simulink model "motorcycle_LQR_with_integral_action"  (R2021a)
settings: Solver=VariableStepAuto  StartTime=0.0  StopTime=10  RelTol=1e-3
values from neighbouring files (symbols this model uses):
  A = [0 0;1 0]    [pole_placement.m]
  B = [1; 0]    [pole_placement.m]
  C = [0 1]    [pole_placement.m]
  k = place(A,B,P)    [pole_placement.m]
undefined symbols (not defined in the file or in its folder): L, L_tK
libraries: simulink x2
settings Model: Creator=martina.elle  LastModifiedBy=francesco

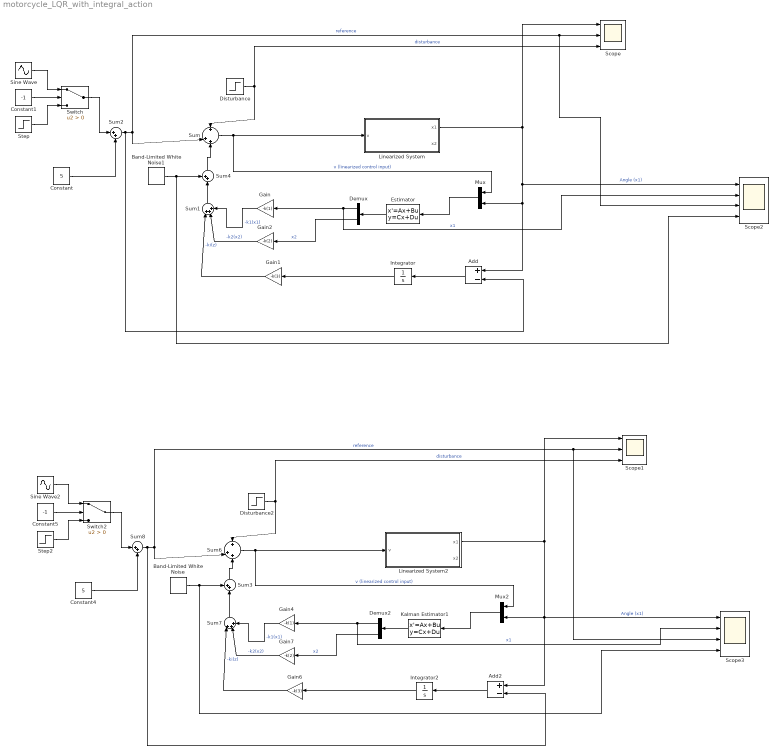
== system motorcycle_LQR_with_integral_action ==
  Add : Sum  Inputs=+-
  Add2 : Sum  Inputs=+-
  Band-Limited White Noise : simulink/Sources/Band-Limited White Noise  Cov=[1]  Ts=0.1  seed=[23341]
  Band-Limited White Noise1 : simulink/Sources/Band-Limited White Noise  Cov=[1]  Ts=0.1  seed=[23341]
  Constant : Constant  Value=5
  Constant1 : Constant  Value=-1
  Constant4 : Constant  Value=5
  Constant5 : Constant  Value=-1
  Demux : Demux  Outputs=2
  Demux2 : Demux  Outputs=2
  Disturbance : Step  After=3  SampleTime=0
  Disturbance2 : Step  After=3  SampleTime=0
  Estimator : StateSpace  A=A-L*C  B=[B L]  C=eye(2)  D=[0 0; 0 0]  InitialCondition=[0 0]  ParameterTunability=Unconstrained
  Gain : Gain  Gain=-k(1)
  Gain1 : Gain  Gain=-k(3)
  Gain2 : Gain  Gain=-k(2)
  Gain4 : Gain  Gain=-k(1)
  Gain6 : Gain  Gain=-k(3)
  Gain7 : Gain  Gain=-k(2)
  Integrator : Integrator  InitialCondition=-3
  Integrator2 : Integrator  InitialCondition=-3
  Kalman Estimator1 : StateSpace  A=A-L_tK*C  B=[B L_tK]  C=eye(2)  D=[0 0; 0 0]  InitialCondition=[0 0]  ParameterTunability=Unconstrained
  Linearized System : Subsystem
  Linearized System2 : Subsystem
  Mux : Mux  Inputs=2
  Mux2 : Mux  Inputs=2
  Scope : Scope  NumInputPorts=3
  Scope1 : Scope  NumInputPorts=3
  Scope2 : Scope  NumInputPorts=4
  Scope3 : Scope  NumInputPorts=4
  Sine Wave : Sin  Frequency=0.1  SampleTime=0
  Sine Wave2 : Sin  Frequency=0.1  SampleTime=0
  Step : Step  After=40  SampleTime=0
  Step2 : Step  After=40  SampleTime=0
  Sum : Sum  Inputs=+|++
  Sum1 : Sum  Inputs=|+++
  Sum2 : Sum  Inputs=|++
  Sum3 : Sum  Inputs=++|
  Sum4 : Sum  Inputs=++|
  Sum6 : Sum  Inputs=+|++
  Sum7 : Sum  Inputs=|+++
  Sum8 : Sum  Inputs=|++
  Switch : Switch  Criteria=u2 > Threshold
  Switch2 : Switch  Criteria=u2 > Threshold
  wires:
  Linearized System/1(x1) -> Mux/2, Add/1, Scope2/1, Scope/1  "Angle (x1)"
  Sum2/1 -> Sum/2, Scope2/3, Scope/2, Add/2  "reference"
  Sum/1 -> Linearized System/1("v "), Mux/1  "v (linearized control input)"
  Mux/1 -> Estimator/1
  Estimator/1 -> Demux/1
  Gain/1 -> Sum1/3  "-k1(x1)"
  Demux/2 -> Gain2/1  "x2"
  Gain2/1 -> Sum1/2  "-k2(x2)"
  Switch/1 -> Sum2/1
  Constant/1 -> Sum2/2
  Constant1/1 -> Switch/2
  Sine Wave/1 -> Switch/1
  Step/1 -> Switch/3
  Gain1/1 -> Sum1/1  "-ki(z)"
  Add/1 -> Integrator/1
  Integrator/1 -> Gain1/1
  Disturbance/1 -> Sum/1, Scope/3  "disturbance"
  Gain4/1 -> Sum7/3  "-k1(x1)"
  Step2/1 -> Switch2/3
  Linearized System2/1(x1) -> Add2/1, Scope3/1, Mux2/2, Scope1/1  "Angle (x1)"
  Sine Wave2/1 -> Switch2/1
  Gain7/1 -> Sum7/2  "-k2(x2)"
  Kalman Estimator1/1 -> Demux2/1
  Switch2/1 -> Sum8/1
  Constant5/1 -> Switch2/2
  Disturbance2/1 -> Sum6/1, Scope1/3  "disturbance"
  Mux2/1 -> Kalman Estimator1/1
  Sum6/1 -> Linearized System2/1("v "), Mux2/1  "v (linearized control input)"
  Constant4/1 -> Sum8/2
  Sum8/1 -> Sum6/2, Scope3/3, Scope1/2, Add2/2  "reference"
  Demux2/2 -> Gain7/1  "x2"
  Demux2/1 -> Scope3/2, Gain4/1  "x1"
  Integrator2/1 -> Gain6/1
  Add2/1 -> Integrator2/1
  Gain6/1 -> Sum7/1  "-ki(z)"
  Band-Limited White Noise/1 -> Scope3/4, Sum3/1
  Sum7/1 -> Sum3/2
  Sum3/1 -> Sum6/3
  Band-Limited White Noise1/1 -> Scope2/4, Sum4/1
  Sum4/1 -> Sum/3
  Sum1/1 -> Sum4/2
  Demux/1 -> Scope2/2, Gain/1  "x1"

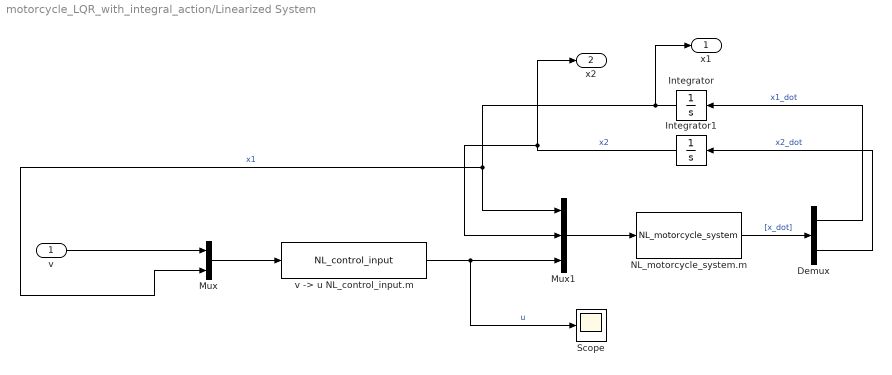
== system motorcycle_LQR_with_integral_action/Linearized System ==
  "v " : Inport
  Demux : Demux  Outputs=2
  Integrator : Integrator  InitialCondition=5
  Integrator1 : Integrator
  Mux : Mux  Inputs=2
  Mux1 : Mux  Inputs=3
  NL_motorcycle_system.m : MATLABFcn  MATLABFcn=NL_motorcycle_system  OutputDimensions=2
  Scope : Scope
  "v -> u NL_control_input.m" : MATLABFcn  MATLABFcn=NL_control_input  OutputDimensions=1
  x1 : Outport
  x2 : Outport  Port=2
  wires:
  Integrator1/1 -> x2/1, Mux1/2  "x2"
  Mux/1 -> "v -> u NL_control_input.m"/1
  "v "/1 -> Mux/1
  Demux/1 -> Integrator/1  "x1_dot"
  Demux/2 -> Integrator1/1  "x2_dot"
  NL_motorcycle_system.m/1 -> Demux/1  "[x_dot]"
  Mux1/1 -> NL_motorcycle_system.m/1
  Integrator/1 -> x1/1, Mux/2, Mux1/1  "x1"
  "v -> u NL_control_input.m"/1 -> Scope/1, Mux1/3  "u"

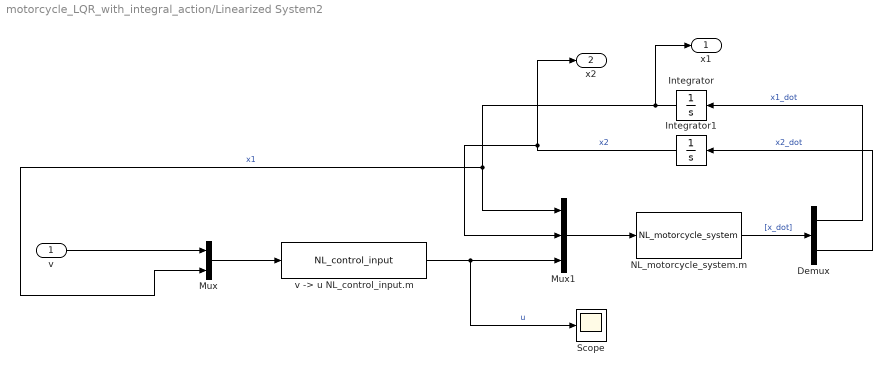
== system motorcycle_LQR_with_integral_action/Linearized System2 ==
  "v " : Inport
  Demux : Demux  Outputs=2
  Integrator : Integrator  InitialCondition=5
  Integrator1 : Integrator
  Mux : Mux  Inputs=2
  Mux1 : Mux  Inputs=3
  NL_motorcycle_system.m : MATLABFcn  MATLABFcn=NL_motorcycle_system  OutputDimensions=2
  Scope : Scope
  "v -> u NL_control_input.m" : MATLABFcn  MATLABFcn=NL_control_input  OutputDimensions=1
  x1 : Outport
  x2 : Outport  Port=2
  wires:
  Integrator1/1 -> x2/1, Mux1/2  "x2"
  NL_motorcycle_system.m/1 -> Demux/1  "[x_dot]"
  "v "/1 -> Mux/1
  Demux/2 -> Integrator1/1  "x2_dot"
  Mux1/1 -> NL_motorcycle_system.m/1
  Mux/1 -> "v -> u NL_control_input.m"/1
  Demux/1 -> Integrator/1  "x1_dot"
  Integrator/1 -> x1/1, Mux/2, Mux1/1  "x1"
  "v -> u NL_control_input.m"/1 -> Scope/1, Mux1/3  "u"
